simulink model "boost_unbalance_trial"  (R2021a)
settings: Solver=FixedStepDiscrete  StartTime=0.0  StopTime=0.2  FixedStep=sampleTime  MaxStep=1e-4  RelTol=1e-4  EnableMultiTasking=on
InitFcn:
  | unbalance_boost
model workspace (MAT data in the model file):
  Phase1 = 0
values from neighbouring files (symbols this model uses):
  CoutModulesp = 271e-6    (= 0.000271)    [boost_parameters.m]    (also in unbalance_boost.m)
  D1 = D+DeltaD    (= 0.25)    [unbalance_boost.m]
  D2 = D-DeltaD    (= 0.25)    [unbalance_boost.m]
  Lcoilsp = 0.517e-3    (= 0.000517)    [boost_parameters.m]    (also in unbalance_boost.m = 0.001034)
  ModuleAPhase = 0    [boost_parameters.m]    (also in flying_capacitor_parameters.m = 90; unbalance_boost.m)
  ModuleBPhase = 180    [boost_parameters.m]    (also in flying_capacitor_parameters.m = 270; unbalance_boost.m)
  Rcoil = 1e-3    (= 0.001)    [boost_parameters.m]    (also in unbalance_boost.m)
  sampleTime = 5e-7    (= 5e-07)    [boost_parameters.m]    (also in flying_capacitor_parameters.m; unbalance_boost.m = 5e-08)
  Vin = 900    [boost_parameters.m]    (also in flying_capacitor_parameters.m; main.m = 880; unbalance_boost.m)
libraries: spsCurrentMeasurementLib x6, spsVoltageMeasurementLib x5, spsSeriesRLCBranchLib x4, dspstat3 x4, simulink x4, spsDiodeLib x2, spsIGBTDiodeLib x2, spsTriangleGeneratorLib x2, spsVariableResistorLib x2, spsDCVoltageSourceLib x1, spspowerguiLib x1
settings Model: Creator=The MathWorks, Inc.  LastModifiedBy=enes_
settings SolverCC: AlgebraicLoopSolver=TrustRegion  SolverResetMethod=Robust
settings OptimizationCC: EfficientFloat2IntCast=on  LifeSpan=inf
settings DebuggingCC: ReadBeforeWriteMsg=DisableAll  WriteAfterWriteMsg=DisableAll  WriteAfterReadMsg=DisableAll  UniqueDataStoreMsg=error  StrictBusMsg=ErrorOnBusTreatedAsVector  SFUnexpectedBacktrackingDiag=warning  SFNoUnconditionalDefaultTransitionDiag=warning  SFExecutionAtInitializationDiag=none  SFMachineParentedDataDiag=warning  ArithmeticOperatorsInVariantConditions=warning
settings ModelReferenceCC: UpdateModelReferenceTargets=IfOutOfDate
settings SFSimCC: SFSimEcho=off  SimUseLocalCustomCode=off  CustomCodeUndefinedFunction=UseInterfaceOnly
settings RTWCC: RTWUseLocalCustomCode=off
settings CodeAppCC: StateflowObjectComments=on
settings GRTTargetCC: TargetLangStandard=C89/C90 (ANSI)
settings ConfigComp: CovMetricSettings=dw  CovSaveCumulativeToWorkspaceVar=on  CovSaveSingleToWorkspaceVar=on  CovExternalEMLEnable=off
settings SimscapeCC: SimscapeNormalizeSystem=off  SimscapeNominalValues={1, 'bar'; 1, 'cm^3/s'; 1, 'bar*kg/s'; 1, 'kJ/kg'; 1, 'kW'; }

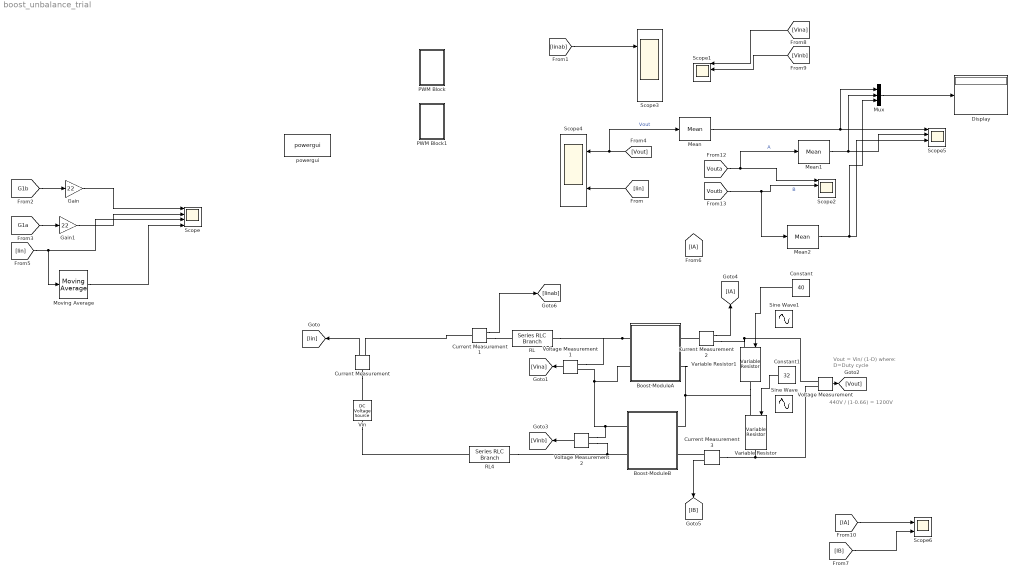
== system boost_unbalance_trial ==
  note: Vout = Vin/ (1-D)
      | where: D=Duty cycle
  note: 440V / (1-0.66) = 1200V
  Boost-ModuleA : Subsystem
  Boost-ModuleB : Subsystem
  Constant : Constant  Value=40
  Constant1 : Constant  Value=32
  Current Measurement{,1..3} (4 alike) : spsCurrentMeasurementLib/Current Measurement  PhasorSimulation=off  OutputType=Complex  PSBequivalent=0
  Display : Display
  Gain : Gain  Gain=22
  Gain1 : Gain  Gain=22
  Mean : dspstat3/Mean  run=on  InputProcessing=Columns as channels (frame based)  reset_popup=None  directionMode=Each column  dimension=1  roiEnable=off  roiType=Rectangles  roiPortion=Entire ROI  roiOutput=Individual statistics for each ROI  roiFlag=off  roundingMode=Floor  overflowMode=off  outputDataTypeStr=Inherit: Same as accumulator  outputMin=[]  outputMax=[]  outputLastDataTypeStr=Inherit: Same as accumulator
  Mean1 : dspstat3/Mean  run=on  InputProcessing=Columns as channels (frame based)  reset_popup=None  directionMode=Each column  dimension=1  roiEnable=off  roiType=Rectangles  roiPortion=Entire ROI  roiOutput=Individual statistics for each ROI  roiFlag=off  roundingMode=Floor  overflowMode=off  outputDataTypeStr=Inherit: Same as accumulator  outputMin=[]  outputMax=[]  outputLastDataTypeStr=Inherit: Same as accumulator
  Mean2 : dspstat3/Mean  run=on  InputProcessing=Columns as channels (frame based)  reset_popup=None  directionMode=Each column  dimension=1  roiEnable=off  roiType=Rectangles  roiPortion=Entire ROI  roiOutput=Individual statistics for each ROI  roiFlag=off  roundingMode=Floor  overflowMode=off  outputDataTypeStr=Inherit: Same as accumulator  outputMin=[]  outputMax=[]  outputLastDataTypeStr=Inherit: Same as accumulator
  Moving Average : dspstat3/Moving Average  Method=Sliding window  ForgettingFactorPort=off  SpecifyWindowLength=on  WindowLength=1/sampleTime/fsw  ForgettingFactor=0.9  SimulateUsing=Code generation
  Mux : Mux  Inputs=3
  PWM Block : Subsystem
  PWM Block1 : Subsystem
  RL : spsSeriesRLCBranchLib/Series RLC Branch  LConnTagsString=__new0  RConnTagsString=__new0  BranchType=L  Resistance=Rcoil  Inductance=Lcoilsp  SetiL0=off  InitialCurrent=8  Capacitance=1e-6  Setx0=off  InitialVoltage=0  Measurements=None
  RL4 : spsSeriesRLCBranchLib/Series RLC Branch  LConnTagsString=__new0  RConnTagsString=__new0  BranchType=L  Resistance=Rcoil  Inductance=Lcoilsp  SetiL0=off  InitialCurrent=8  Capacitance=1e-6  Setx0=off  InitialVoltage=0  Measurements=None
  Scope{,1..2,5} (4 alike) : Scope  NumInputPorts=4
  Scope3 : Scope  NumInputPorts=2
  Scope4 : Scope  NumInputPorts=2
  Scope6 : Scope  NumInputPorts=2
  Sine Wave : Sin  Bias=36  Frequency=150*2*pi  SampleTime=0
  Sine Wave1 : Sin  Bias=36  Frequency=150*2*pi  Phase=pi  SampleTime=0
  Variable Resistor : spsVariableResistorLib/Variable Resistor  Rabsmin=1e-3
      settings: SourceProductBaseCode=PS
  Variable Resistor1 : spsVariableResistorLib/Variable Resistor  Rabsmin=1e-3
      settings: SourceProductBaseCode=PS
  "Vin   " : spsDCVoltageSourceLib/DC Voltage Source  Amplitude=Vin  Measurements=None
  Voltage Measurement : spsVoltageMeasurementLib/Voltage Measurement  PhasorSimulation=off  OutputType=Complex  PSBequivalent=0
  Voltage Measurement1 : spsVoltageMeasurementLib/Voltage Measurement  PhasorSimulation=off  OutputType=Complex  PSBequivalent=0
  Voltage Measurement2 : spsVoltageMeasurementLib/Voltage Measurement  PhasorSimulation=off  OutputType=Complex  PSBequivalent=0
  powergui : spspowerguiLib/powergui  Priority=1  SimulationMode=Discrete  SampleTime=sampleTime  frequency=60  Iterations=50  frequencyindice=0  Pbase=100e6  ErrMax=1e-4  UnitsV=kV  UnitsW=MW  buscounter=0  FunctionMessages=off  echomessages=off  EnableUseOfTLC=off  CurrentSourceSwitches=off  DisableSnubberDevices=off  DisableRonSwitches=off  DisableVfSwitches=off  DisplayEquations=off  AutomaticDiscreteSolvers=off  SolverType=Tustin/Backward Euler (TBE)  Interpol=off  ExternalGateDelay=off  methode=off  Ts=100  x0status=blocks  SPID=on  SwTol=0  HookPort=off  NonlinearTolerance=1e-4  nMaxIteration=100  ContinueOnMaxIteration=off  RestoreLinks=warning  ResistiveCurrentMeasurement=off  Frange=[0:2:500]  Ylog=off  Xlog=on  ShowGrid=off  save=off  variable=ZData  structure=0  ZoomFFT=off  StartTime=0.0  cycles=1  DisplayStyle=1  fundamental=60  FreqAxis=off  MaxFrequency=1000  frequencyindicesteady=1  RmsSteady=1  display=off
  wires:
  [Vout] -> Mean/1, Scope4/1  "Vout"
  [Iin] -> Scope4/2
  [Vina] -> Scope1/1
  [Vinb] -> Scope1/2
  ? -> Scope1/3
  ? -> Scope1/4
  ? -> Scope3/2
  [Iinab] -> Scope3/1
  [Vouta] -> Mean1/1, Scope2/1  "A"
  [Voutb] -> Mean2/1, Scope2/2  "B"
  Current Measurement1/1 -> [Iinab]
  Voltage Measurement2/1 -> [Vinb]
  Voltage Measurement1/1 -> [Vina]
  Current Measurement/1 -> [Iin]
  Voltage Measurement/1 -> [Vout]
  Constant/1 -> Variable Resistor1/1
  Constant1/1 -> Variable Resistor/1
  Mean/1 -> Mux/1, Scope5/1
  Mean1/1 -> Mux/2, Scope5/2
  Mean2/1 -> Mux/3, Scope5/3
  Mux/1 -> Display/1
  [G1b] -> Gain/1
  [G1a] -> Gain1/1
  Gain/1 -> Scope/1
  Gain1/1 -> Scope/2
  [Iin] -> Moving Average/1, Scope/3
  Current Measurement2/1 -> [IA]
  Current Measurement3/1 -> [IB]
  [IA] -> Scope6/1
  [IB] -> Scope6/2
  Moving Average/1 -> Scope/4
  connections:
  Boost-ModuleA/RConn2 -- Variable Resistor1/RConn1 -- Variable Resistor/LConn1 -- Boost-ModuleB/RConn1
  Current Measurement1/RConn1 -- RL/LConn1
  Boost-ModuleA/LConn1 -- RL/RConn1 -- Voltage Measurement1/LConn1
  Current Measurement1/LConn1 -- Current Measurement/RConn1
  Current Measurement3/LConn1 -- Voltage Measurement/LConn2 -- Variable Resistor/RConn1
  Boost-ModuleA/LConn2 -- Voltage Measurement2/LConn1 -- Boost-ModuleB/LConn1 -- Voltage Measurement1/LConn2
  Voltage Measurement2/LConn2 -- RL4/RConn1 -- Boost-ModuleB/LConn2
  Voltage Measurement/LConn1 -- Current Measurement2/RConn1 -- Variable Resistor1/LConn1
  Current Measurement/LConn1 -- "Vin   "/RConn1
  "Vin   "/LConn1 -- RL4/LConn1
  Current Measurement2/LConn1 -- Boost-ModuleA/RConn1
  Current Measurement3/RConn1 -- Boost-ModuleB/RConn2

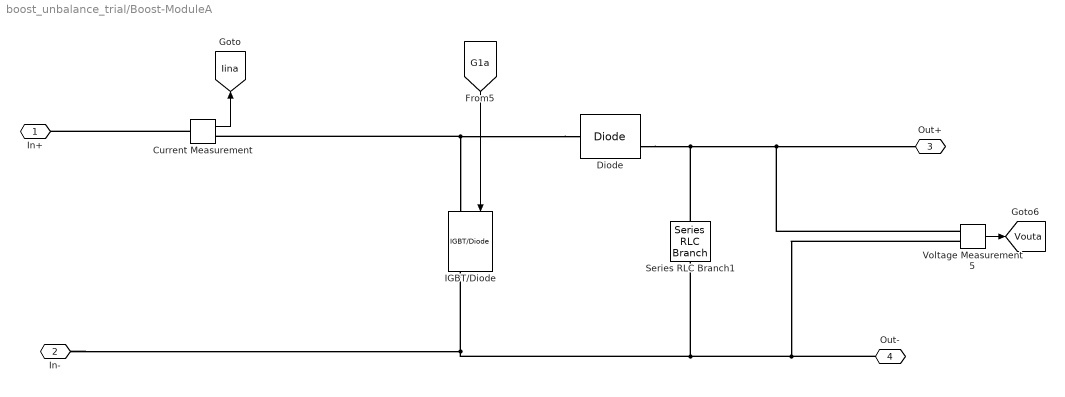
== system boost_unbalance_trial/Boost-ModuleA ==
  Current Measurement : spsCurrentMeasurementLib/Current Measurement  PhasorSimulation=off  OutputType=Complex  PSBequivalent=0
  Diode : spsDiodeLib/Diode  Ron=0.001  Lon=0  Vf=0.8  IC=0  UseSnubber=0  Rs=500  Cs=250e-9  Measurements=on
  IGBT/Diode : spsIGBTDiodeLib/IGBT//Diode  Ron=1e-3  Rs=1e5  Cs=inf  Measurements=on
  Series RLC Branch1 : spsSeriesRLCBranchLib/Series RLC Branch  LConnTagsString=__new0  RConnTagsString=__new0  BranchType=C  Resistance=1e-4  Inductance=200e-6  SetiL0=off  InitialCurrent=0  Capacitance=CoutModulesp  Setx0=off  InitialVoltage=1200  Measurements=None
  Voltage Measurement5 : spsVoltageMeasurementLib/Voltage Measurement  PhasorSimulation=off  OutputType=Complex  PSBequivalent=0
  In+ : PMIOPort  Side=Left
  In- : PMIOPort  Port=2  Side=Left
  Out+ : PMIOPort  Port=3  Side=Right
  Out- : PMIOPort  Port=4  Side=Right
  tag scope: Iina=global, Vouta=global
  wires:
  [G1a] -> IGBT/Diode/1
  Current Measurement/1 -> [Iina]
  Voltage Measurement5/1 -> [Vouta]
  connections:
  Diode/LConn1 -- IGBT/Diode/LConn1 -- Current Measurement/RConn1
  Series RLC Branch1/LConn1 -- Diode/RConn1 -- Voltage Measurement5/LConn1 -- Out+/RConn1
  Current Measurement/LConn1 -- In+/RConn1
  Out-/RConn1 -- Voltage Measurement5/LConn2 -- In-/RConn1 -- IGBT/Diode/RConn1 -- Series RLC Branch1/RConn1

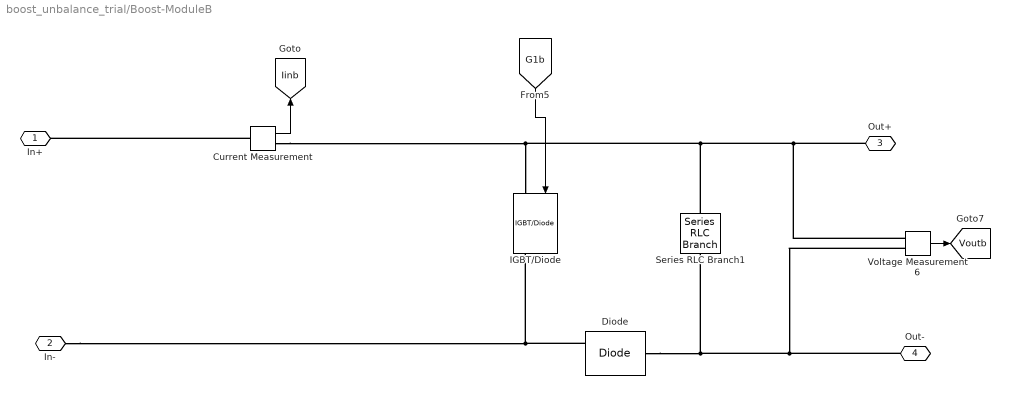
== system boost_unbalance_trial/Boost-ModuleB ==
  Current Measurement : spsCurrentMeasurementLib/Current Measurement  PhasorSimulation=off  OutputType=Complex  PSBequivalent=0
  Diode : spsDiodeLib/Diode  Ron=0.001  Lon=0  Vf=0.8  IC=0  UseSnubber=0  Rs=500  Cs=250e-9  Measurements=on
  IGBT/Diode : spsIGBTDiodeLib/IGBT//Diode  Ron=1e-3  Rs=1e5  Cs=inf  Measurements=on
  Series RLC Branch1 : spsSeriesRLCBranchLib/Series RLC Branch  LConnTagsString=__new0  RConnTagsString=__new0  BranchType=C  Resistance=1e-4  Inductance=200e-6  SetiL0=off  InitialCurrent=0  Capacitance=CoutModulesp  Setx0=off  InitialVoltage=1200  Measurements=None
  Voltage Measurement6 : spsVoltageMeasurementLib/Voltage Measurement  PhasorSimulation=off  OutputType=Complex  PSBequivalent=0
  In+ : PMIOPort  Side=Left
  In- : PMIOPort  Port=2  Side=Left
  Out+ : PMIOPort  Port=3  Side=Right
  Out- : PMIOPort  Port=4  Side=Right
  tag scope: Iinb=global, Voutb=global
  wires:
  Current Measurement/1 -> [Iinb]
  [G1b] -> IGBT/Diode/1
  Voltage Measurement6/1 -> [Voutb]
  connections:
  Out+/RConn1 -- Voltage Measurement6/LConn1 -- Series RLC Branch1/LConn1 -- Current Measurement/RConn1 -- IGBT/Diode/LConn1
  Out-/RConn1 -- Voltage Measurement6/LConn2 -- Diode/LConn1 -- Series RLC Branch1/RConn1
  Current Measurement/LConn1 -- In+/RConn1
  In-/RConn1 -- Diode/RConn1 -- IGBT/Diode/RConn1

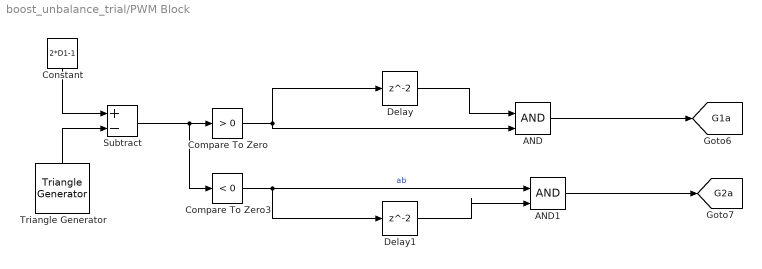
== system boost_unbalance_trial/PWM Block ==
  AND : Logic  IconShape=distinctive  AllPortsSameDT=off  OutDataTypeStr=boolean
  AND1 : Logic  IconShape=distinctive  AllPortsSameDT=off  OutDataTypeStr=boolean
  Compare To Zero : simulink/Logic and Bit Operations/Compare To Zero  relop=>  OutDataTypeStr=boolean
  Compare To Zero3 : simulink/Logic and Bit Operations/Compare To Zero  relop=<  OutDataTypeStr=boolean
  Constant : Constant  Value=2*D1-1
  Delay : Delay
  Delay1 : Delay
  Subtract : Sum  Inputs=+-
  Triangle Generator : spsTriangleGeneratorLib/Triangle Generator  Freq=fsw  Phase=ModuleAPhase  Ts=sampleTime
  tag scope: G1a=global, G2a=global
  wires:
  Constant/1 -> Subtract/1
  Triangle Generator/1 -> Subtract/2
  Subtract/1 -> Compare To Zero3/1, Compare To Zero/1
  AND/1 -> [G1a]
  Compare To Zero/1 -> Delay/1, AND/2
  Delay/1 -> AND/1
  Compare To Zero3/1 -> Delay1/1, AND1/1  "ab"
  AND1/1 -> [G2a]
  Delay1/1 -> AND1/2

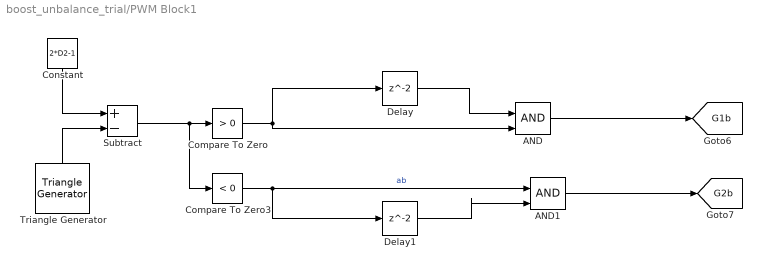
== system boost_unbalance_trial/PWM Block1 ==
  AND : Logic  IconShape=distinctive  AllPortsSameDT=off  OutDataTypeStr=boolean
  AND1 : Logic  IconShape=distinctive  AllPortsSameDT=off  OutDataTypeStr=boolean
  Compare To Zero : simulink/Logic and Bit Operations/Compare To Zero  relop=>  OutDataTypeStr=boolean
  Compare To Zero3 : simulink/Logic and Bit Operations/Compare To Zero  relop=<  OutDataTypeStr=boolean
  Constant : Constant  Value=2*D2-1
  Delay : Delay
  Delay1 : Delay
  Subtract : Sum  Inputs=+-
  Triangle Generator : spsTriangleGeneratorLib/Triangle Generator  Freq=fsw  Phase=ModuleBPhase  Ts=sampleTime
  tag scope: G1b=global, G2b=global
  wires:
  Constant/1 -> Subtract/1
  Triangle Generator/1 -> Subtract/2
  Subtract/1 -> Compare To Zero3/1, Compare To Zero/1
  AND/1 -> [G1b]
  Compare To Zero/1 -> Delay/1, AND/2
  Delay/1 -> AND/1
  Compare To Zero3/1 -> Delay1/1, AND1/1  "ab"
  AND1/1 -> [G2b]
  Delay1/1 -> AND1/2
